simulink model "Time_Shift_1"  (R2015a)
settings: Solver=ode3  StartTime=0.0  StopTime=inf  FixedStep=.1  RelTol=1e-3
libraries: xpcutilitieslib x31, slrtlib x10, AAxpcseriallibold x9, xpcobsoletelib x5, etargetslib x1
settings Model: SimulationMode=external  Creator=farbod  LastModifiedBy=Darryl
settings SolverCC: EnableConcurrentExecution=on
settings DataIOCC: SignalLoggingSaveFormat=ModelDataLogs
settings OptimizationCC: BlockReduction=off  OptimizeBlockIOStorage=off  BufferReuse=off  GlobalBufferReuse=off  ExpressionFolding=off  ExpressionDepthLimit=2147483647  LocalBlockOutputs=off
settings DebuggingCC: UnderspecifiedInitializationDetection=Classic  MergeDetectMultiDrivingBlocksExec=none  FcnCallInpInsideContextMsg=UseLocalSettings  StateNameClashWarn=warning
settings HardwareCC: ProdIntDivRoundTo=Zero  ProdEndianess=LittleEndian  ProdLongLongMode=on  ProdHWDeviceType=Generic->32-bit x86 compatible  TargetBitPerLong=64  TargetBitPerPointer=64  TargetIntDivRoundTo=Zero  TargetEndianess=LittleEndian  TargetWordSize=64  TargetHWDeviceType=Intel->x86-64
settings SFSimCC: SimParseCustomCode=off
settings RTWCC: SystemTargetFile=slrt.tlc  TemplateMakefile=slrt_default_tmf  Description=Simulink Real-Time  RTWVerbose=off  RTWCompilerOptimization=on
settings CodeAppCC: MaxIdLength=95
settings SimulinkRealTimeCC: GeneratePreprocessorConditionals=Disable all

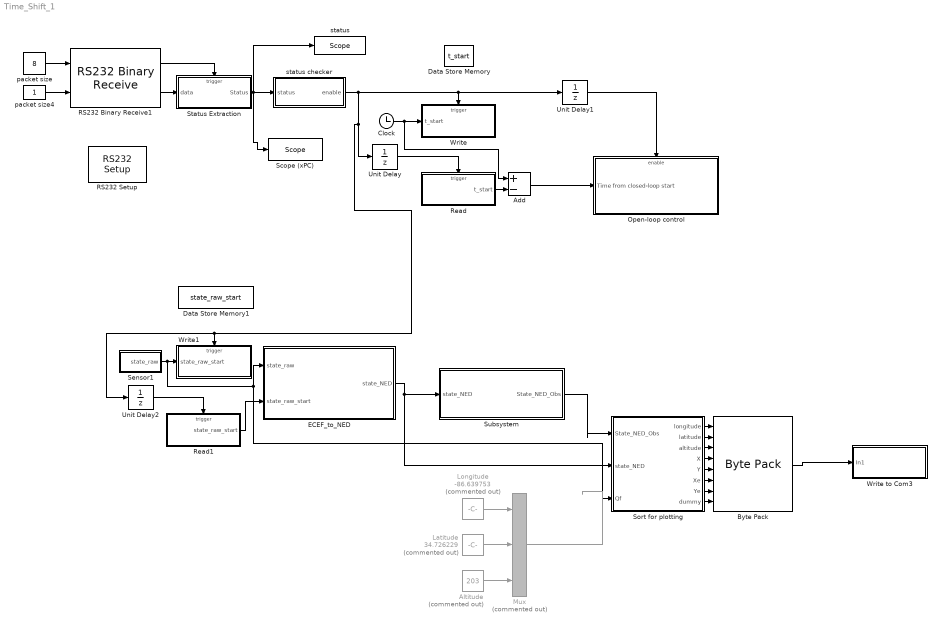
== system Time_Shift_1 ==
  Add : Sum  Inputs=+-
  Altitude : Constant  Commented=on  Value=203
  Byte Pack : etargetslib/Byte Pack  datatypes={'uint8','uint8','uint8','uint8','uint8','uint8','uint8','uint8'}  byteAlign=1
  Clock : Clock
  Data Store Memory : DataStoreMemory  DataStoreName=t_start  ReadBeforeWriteMsg=warning  WriteAfterWriteMsg=warning  WriteAfterReadMsg=warning
  Data Store Memory1 : DataStoreMemory  DataStoreName=state_raw_start  ReadBeforeWriteMsg=warning  WriteAfterWriteMsg=warning  WriteAfterReadMsg=warning  InitialValue=[-86.647163*pi/180;34.718727*pi/180;195;0;0;0;0;0;0;0;0;0;0;0;-1]
  ECEF_to_NED : MATLAB Function  TreatAsAtomicUnit=on
  Latitude : Constant  Commented=on  Value=34.726229
  Longitude : Constant  Commented=on  Value=-86.639753
  Mux : Mux  Commented=on  Inputs=3
  Open-loop control : Subsystem
  RS232 Binary Receive1 : AAxpcseriallibold/Obsolete/Binary Mode/RS232 Binary Receive  port=COM1  width=8  samptime=-1
  "RS232 Setup " : AAxpcseriallibold/Obsolete/RS232 Setup   port=COM1  baud=115200  dbits=8  sbits=1  parity=None  prot=None  sbuf=2048  rbuf=2048  initstruct=[]  termstruct=[]
  Read : Subsystem  TreatAsAtomicUnit=on
  Read1 : Subsystem  TreatAsAtomicUnit=on
  "Scope (xPC) " : slrtlib/Displays and Logging/Scope   scopeno=2  scopetype=Target  autostart=on  viewmode=Graphical rolling  formatstr='status=%3.3f'  grid=on  ylimits=[0,0]  nosamples=2000  noprepostsamples=0  interleave=1  triggermode=FreeRun  triggersignal=1  trigsignalfromport=off  triggerlevel=0.0  triggerslope=Either  triggerscope=1  triggersample=0  filename=data.dat  mode=Lazy  writesize=512  autorestart=off  dynamicfilemode=off  maxwritefilesize=512*1024^2
  Sensor1 : Subsystem
  Sort for plotting : MATLAB Function  TreatAsAtomicUnit=on
  Status Extraction : Subsystem  TreatAsAtomicUnit=on
  Subsystem : Subsystem
  Unit Delay : UnitDelay  SampleTime=-1
  Unit Delay1 : UnitDelay  SampleTime=-1
  Unit Delay2 : UnitDelay  SampleTime=-1
  Write : Subsystem  TreatAsAtomicUnit=on
  Write to Com3 : Subsystem
  Write1 : Subsystem  TreatAsAtomicUnit=on
  packet size : Constant  Value=8
  packet size4 : Constant
  status : slrtlib/Displays and Logging/Scope   scopeno=6  scopetype=File  autostart=on  viewmode=Graphical rolling  formatstr='%15.6f'  grid=on  ylimits=[-10,50]  nosamples=3000  noprepostsamples=0  interleave=1  triggermode=FreeRun  triggersignal=1  trigsignalfromport=off  triggerlevel=0.0  triggerslope=Either  triggerscope=1  triggersample=0  filename=1sttus01.dat  mode=Commit  writesize=512  autorestart=on  dynamicfilemode=off  maxwritefilesize=512*1024^2
  status checker : MATLAB Function  TreatAsAtomicUnit=on
  wires:
  Unit Delay/1 -> Read/Trigger
  Clock/1 -> Write/1(t_start), Add/1
  Read/1(t_start) -> Add/2
  Status Extraction/1(Status) -> status/1, "Scope (xPC) "/1, status checker/1(status)
  status checker/1(enable) -> Write/Trigger, Unit Delay1/1, Unit Delay/1, Unit Delay2/1, Write1/Trigger
  Unit Delay1/1 -> Open-loop control/Enable
  Add/1 -> Open-loop control/1(Time from closed-loop start)
  Sensor1/1(state_raw) -> Write1/1(state_raw_start), Sort for plotting/3(Qf), ECEF_to_NED/1(state_raw)
  Unit Delay2/1 -> Read1/Trigger
  Read1/1(state_raw_start) -> ECEF_to_NED/2(state_raw_start)
  ECEF_to_NED/1(state_NED) -> Sort for plotting/2(state_NED), Subsystem/1(state_NED)
  RS232 Binary Receive1/2 -> Status Extraction/1(data)
  RS232 Binary Receive1/1 -> Status Extraction/Trigger
  packet size4/1 -> RS232 Binary Receive1/2
  packet size/1 -> RS232 Binary Receive1/1
  Subsystem/1(State_NED_Obs) -> Sort for plotting/1(State_NED_Obs)
  Latitude/1 -> Mux/2
  Altitude/1 -> Mux/3
  Longitude/1 -> Mux/1
  Mux/1 -> ?
  Byte Pack/1 -> Write to Com3/1(In1)
  Sort for plotting/1(longitude) -> Byte Pack/1
  Sort for plotting/2(latitude) -> Byte Pack/2
  Sort for plotting/3(altitude) -> Byte Pack/3
  Sort for plotting/4(X) -> Byte Pack/4
  Sort for plotting/5(Y) -> Byte Pack/5
  Sort for plotting/6(Xe) -> Byte Pack/6
  Sort for plotting/7(Ye) -> Byte Pack/7
  Sort for plotting/8(dummy) -> Byte Pack/8

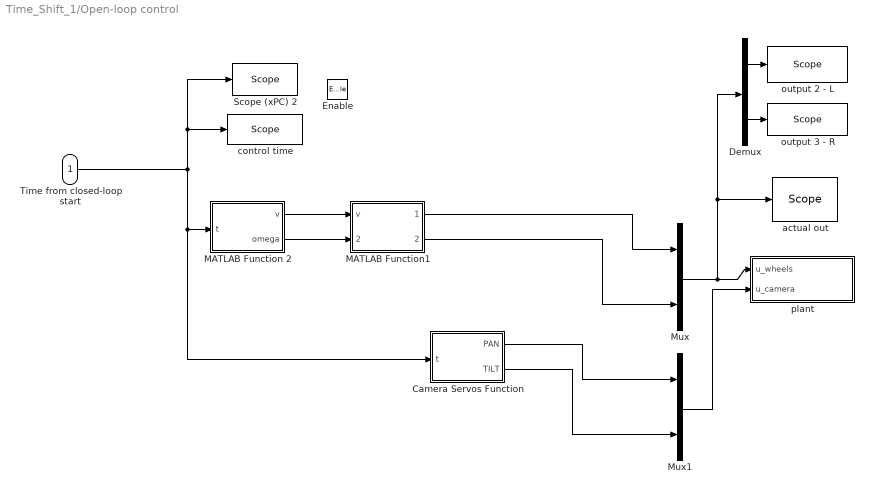
== system Time_Shift_1/Open-loop control ==
  Time from closed-loop start : Inport
  Enable : EnablePort  PropagateVarSize=During execution
  " MATLAB Function1" : MATLAB Function  TreatAsAtomicUnit=on
  Camera Servos Function : MATLAB Function  TreatAsAtomicUnit=on
  Demux : Demux  Outputs=2
  MATLAB Function 2 : MATLAB Function  TreatAsAtomicUnit=on
  Mux : Mux  Inputs=2
  Mux1 : Mux  Inputs=2
  Scope (xPC) 2 : slrtlib/Displays and Logging/Scope   scopeno=1  scopetype=File  autostart=on  viewmode=Graphical redraw  formatstr='%15.6f'  grid=on  ylimits=[0,0]  nosamples=3000  noprepostsamples=0  interleave=1  triggermode=FreeRun  triggersignal=1  trigsignalfromport=off  triggerlevel=0.0  triggerslope=Either  triggerscope=1  triggersample=0  filename=1ctime01.dat  mode=Commit  writesize=512  autorestart=off  dynamicfilemode=off  maxwritefilesize=512*1024^2
  actual out : slrtlib/Displays and Logging/Scope   scopeno=7  scopetype=File  autostart=on  viewmode=Graphical rolling  formatstr='%15.6f'  grid=on  ylimits=[-3,150]  nosamples=3000  noprepostsamples=0  interleave=1  triggermode=FreeRun  triggersignal=1  trigsignalfromport=off  triggerlevel=0.0  triggerslope=Either  triggerscope=1  triggersample=0  filename=1pwm01.dat  mode=Commit  writesize=512  autorestart=on  dynamicfilemode=off  maxwritefilesize=512*1024^2
  control time : slrtlib/Displays and Logging/Scope   scopeno=9  scopetype=Target  autostart=on  viewmode=Graphical rolling  formatstr='t=%3.3f'  grid=on  ylimits=[0,0]  nosamples=2000  noprepostsamples=0  interleave=1  triggermode=FreeRun  triggersignal=1  trigsignalfromport=off  triggerlevel=0.0  triggerslope=Either  triggerscope=1  triggersample=0  filename=data.dat  mode=Lazy  writesize=512  autorestart=off  dynamicfilemode=off  maxwritefilesize=512*1024^2
  output 2 - L : slrtlib/Displays and Logging/Scope   scopeno=10  scopetype=Target  autostart=on  viewmode=Graphical rolling  formatstr='u1=%3.3f'  grid=on  ylimits=[0,0]  nosamples=20000  noprepostsamples=0  interleave=1  triggermode=FreeRun  triggersignal=1  trigsignalfromport=off  triggerlevel=0.0  triggerslope=Either  triggerscope=1  triggersample=0  filename=data.dat  mode=Lazy  writesize=512  autorestart=off  dynamicfilemode=off  maxwritefilesize=512*1024^2
  output 3 - R : slrtlib/Displays and Logging/Scope   scopeno=5  scopetype=Target  autostart=on  viewmode=Graphical rolling  formatstr='u2=%3.3f'  grid=on  ylimits=[0,0]  nosamples=20000  noprepostsamples=0  interleave=1  triggermode=FreeRun  triggersignal=1  trigsignalfromport=off  triggerlevel=0.0  triggerslope=Either  triggerscope=1  triggersample=0  filename=data.dat  mode=Lazy  writesize=512  autorestart=off  dynamicfilemode=off  maxwritefilesize=512*1024^2
  plant : Subsystem
  wires:
  Time from closed-loop start/1 -> control time/1, Scope (xPC) 2/1, MATLAB Function 2/1(t), Camera Servos Function/1(t)
  Demux/1 -> output 2 - L/1
  Demux/2 -> output 3 - R/1
  Mux/1 -> plant/1(u_wheels), actual out/1, Demux/1
  MATLAB Function 2/1(v) -> " MATLAB Function1"/1(v)
  MATLAB Function 2/2(omega) -> " MATLAB Function1"/2(omega)
  " MATLAB Function1"/1(PWM_L) -> Mux/1
  " MATLAB Function1"/2(PWM_R) -> Mux/2
  Camera Servos Function/1(PAN) -> Mux1/1
  Camera Servos Function/2(TILT) -> Mux1/2
  Mux1/1 -> plant/2(u_camera)

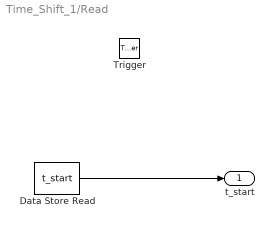
== system Time_Shift_1/Read ==
  Trigger : TriggerPort
  Data Store Read : DataStoreRead  DataStoreName=t_start
  t_start : Outport
  wires:
  Data Store Read/1 -> t_start/1

== system Time_Shift_1/Read1 ==
  Trigger : TriggerPort
  Data Store Read : DataStoreRead  DataStoreName=state_raw_start
  state_raw_start : Outport
  wires:
  Data Store Read/1 -> state_raw_start/1

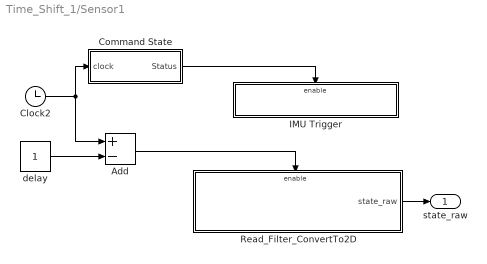
== system Time_Shift_1/Sensor1 ==
  Add : Sum  Inputs=+-
  Clock2 : Clock
  Command State : MATLAB Function  TreatAsAtomicUnit=on
  IMU Trigger : Subsystem
  Read_Filter_ConvertTo2D : Subsystem
  delay : Constant
  state_raw : Outport
  wires:
  Clock2/1 -> Add/1, Command State/1(clock)
  Read_Filter_ConvertTo2D/1(state_raw) -> state_raw/1
  delay/1 -> Add/2
  Add/1 -> Read_Filter_ConvertTo2D/Enable
  Command State/1(Status) -> IMU Trigger/Enable

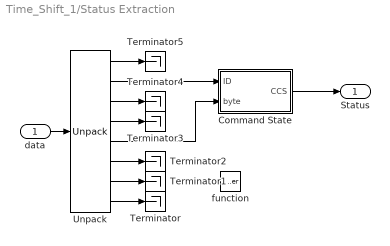
== system Time_Shift_1/Status Extraction ==
  data : Inport
  function : TriggerPort  TriggerType=function-call  OutputDataType=int8
  Command State : MATLAB Function  TreatAsAtomicUnit=on
  Terminator{,1..5} (6 alike) : Terminator
  Unpack : xpcobsoletelib/Utilities/Unpack   dimensions={1,1,1,1,1,1,1,1}  datatypes={'uint8','uint8','uint8','uint8','uint8','uint8','uint8','uint8'}  byteAlign=1
  Status : Outport
  wires:
  data/1 -> Unpack/1
  Command State/1(CCS) -> Status/1
  Unpack/5 -> Command State/2(byte)
  Unpack/2 -> Command State/1(ID)
  Unpack/8 -> Terminator/1
  Unpack/1 -> Terminator5/1
  Unpack/3 -> Terminator4/1
  Unpack/4 -> Terminator3/1
  Unpack/6 -> Terminator2/1
  Unpack/7 -> Terminator1/1

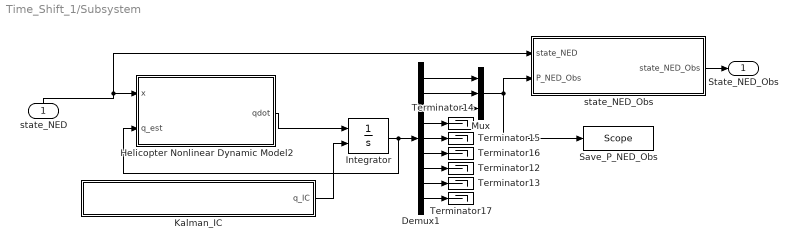
== system Time_Shift_1/Subsystem ==
  state_NED : Inport
  Demux1 : Demux  Outputs=9
  Helicopter Nonlinear Dynamic Model2 : MATLAB Function  TreatAsAtomicUnit=on
  Integrator : Integrator  InitialConditionSource=external
  Kalman_IC : MATLAB Function  TreatAsAtomicUnit=on
  Mux : Mux  Inputs=3
  Save_P_NED_Obs : slrtlib/Displays and Logging/Scope   scopeno=4  scopetype=File  autostart=on  viewmode=Graphical rolling  formatstr='%15.6f'  grid=on  ylimits=[-10,50]  nosamples=3000  noprepostsamples=0  interleave=1  triggermode=FreeRun  triggersignal=1  trigsignalfromport=off  triggerlevel=0.0  triggerslope=Either  triggerscope=1  triggersample=0  filename=1P_NED1.dat  mode=Commit  writesize=512  autorestart=on  dynamicfilemode=off  maxwritefilesize=512*1024^2
  Terminator{12..17} (6 alike) : Terminator
  state_NED_Obs : MATLAB Function  TreatAsAtomicUnit=on
  State_NED_Obs : Outport
  wires:
  state_NED/1 -> state_NED_Obs/1(state_NED), Helicopter Nonlinear Dynamic Model2/1(x)
  Integrator/1 -> Demux1/1, Helicopter Nonlinear Dynamic Model2/2(q_est)
  Kalman_IC/1(q_IC) -> Integrator/2
  Demux1/4 -> Terminator14/1
  Demux1/5 -> Terminator15/1
  Demux1/6 -> Terminator16/1
  Demux1/7 -> Terminator12/1
  Demux1/8 -> Terminator13/1
  Demux1/9 -> Terminator17/1
  Helicopter Nonlinear Dynamic Model2/1(qdot) -> Integrator/1
  Demux1/3 -> Mux/3
  Demux1/2 -> Mux/2
  Demux1/1 -> Mux/1
  Mux/1 -> state_NED_Obs/2(P_NED_Obs), Save_P_NED_Obs/1
  state_NED_Obs/1(state_NED_Obs) -> State_NED_Obs/1

== system Time_Shift_1/Write ==
  t_start : Inport
  Trigger : TriggerPort
  Data Store Write : DataStoreWrite  DataStoreName=t_start
  wires:
  t_start/1 -> Data Store Write/1

== system Time_Shift_1/Write to Com3 ==
  In1 : Inport
  RS232 Binary Send : AAxpcseriallibold/Obsolete/Binary Mode/RS232 Binary Send  port=COM3  width=64  samptime=-1
  "RS232 Setup " : AAxpcseriallibold/Obsolete/RS232 Setup   port=COM3  baud=19200  dbits=8  sbits=1  parity=None  prot=XOn XOff  sbuf=960000  rbuf=2048  initstruct=[]  termstruct=[]
  wires:
  In1/1 -> RS232 Binary Send/1

== system Time_Shift_1/Write1 ==
  state_raw_start : Inport
  Trigger : TriggerPort
  Data Store Write : DataStoreWrite  DataStoreName=state_raw_start
  wires:
  state_raw_start/1 -> Data Store Write/1

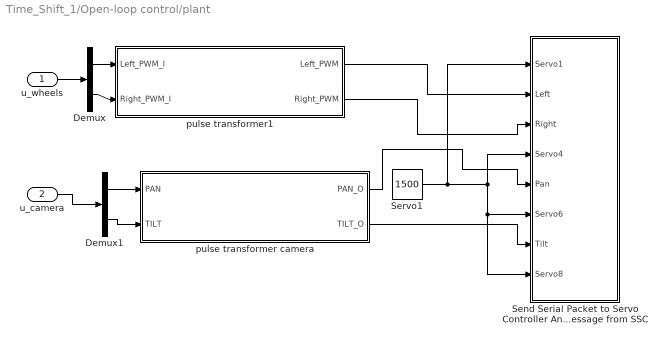
== system Time_Shift_1/Open-loop control/plant ==
  u_wheels : Inport
  u_camera : Inport  Port=2
  Demux : Demux  Outputs=2
  Demux1 : Demux  Outputs=2
  Send Serial Packet to Servo Controller And recieve status message from SSC : Subsystem  TreatAsAtomicUnit=on
  Servo1 : Constant  Value=1500  OutDataTypeStr=uint16
  pulse transformer camera : MATLAB Function  TreatAsAtomicUnit=on
  pulse transformer1 : MATLAB Function  TreatAsAtomicUnit=on
  wires:
  Servo1/1 -> Send Serial Packet to Servo Controller And recieve status message from SSC/6(Servo6), Send Serial Packet to Servo Controller And recieve status message from SSC/8(Servo8), Send Serial Packet to Servo Controller And recieve status message from SSC/4(Servo4), Send Serial Packet to Servo Controller And recieve status message from SSC/1(Servo1)
  u_wheels/1 -> Demux/1
  Demux/1 -> pulse transformer1/1(Left_PWM_I)
  Demux/2 -> pulse transformer1/2(Right_PWM_I)
  u_camera/1 -> Demux1/1
  pulse transformer1/1(Left_PWM) -> Send Serial Packet to Servo Controller And recieve status message from SSC/2(Left)
  pulse transformer1/2(Right_PWM) -> Send Serial Packet to Servo Controller And recieve status message from SSC/3(Right)
  Demux1/1 -> pulse transformer camera/1(PAN)
  Demux1/2 -> pulse transformer camera/2(TILT)
  pulse transformer camera/1(PAN_O) -> Send Serial Packet to Servo Controller And recieve status message from SSC/5(Pan)
  pulse transformer camera/2(TILT_O) -> Send Serial Packet to Servo Controller And recieve status message from SSC/7(Tilt)

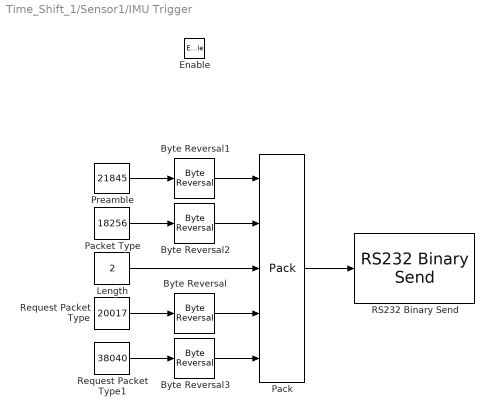
== system Time_Shift_1/Sensor1/IMU Trigger ==
  Enable : EnablePort  PropagateVarSize=During execution
  Byte Reversal{,1..3} (4 alike) : xpcutilitieslib/Byte Reversal   numInp=1
  Length : Constant  Value=2  OutDataTypeStr=uint8
  Pack : xpcobsoletelib/Utilities/Pack   datatypes={'uint16','uint16','uint8','uint16','uint16'}  byteAlign=1
  Packet Type : Constant  Value=18256  OutDataTypeStr=uint16
  Preamble : Constant  Value=21845  OutDataTypeStr=uint16
  RS232 Binary Send : AAxpcseriallibold/Obsolete/Binary Mode/RS232 Binary Send  port=COM2  width=9  samptime=-1
  Request Packet Type : Constant  Value=20017  OutDataTypeStr=uint16
  Request Packet Type1 : Constant  Value=38040  OutDataTypeStr=uint16
  wires:
  Pack/1 -> RS232 Binary Send/1
  Preamble/1 -> Byte Reversal1/1
  Packet Type/1 -> Byte Reversal2/1
  Length/1 -> Pack/3
  Request Packet Type/1 -> Byte Reversal/1
  Request Packet Type1/1 -> Byte Reversal3/1
  Byte Reversal/1 -> Pack/4
  Byte Reversal1/1 -> Pack/1
  Byte Reversal2/1 -> Pack/2
  Byte Reversal3/1 -> Pack/5

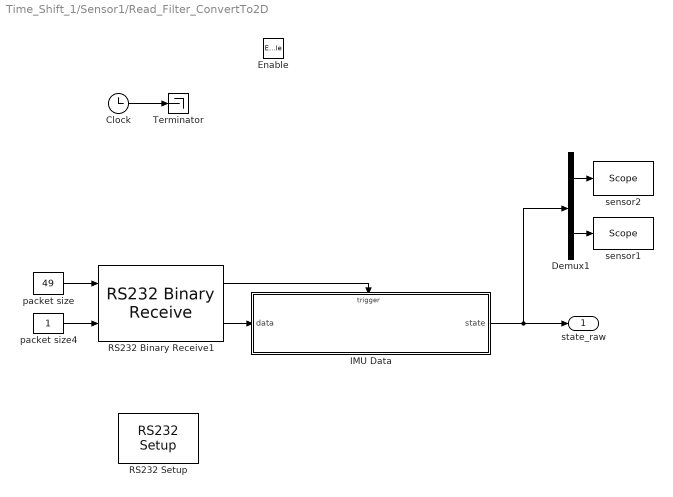
== system Time_Shift_1/Sensor1/Read_Filter_ConvertTo2D ==
  Enable : EnablePort  PropagateVarSize=During execution
  Clock : Clock
  Demux1 : Demux  Outputs=2
  IMU Data : Subsystem  TreatAsAtomicUnit=on
  RS232 Binary Receive1 : AAxpcseriallibold/Obsolete/Binary Mode/RS232 Binary Receive  port=COM2  width=49  samptime=-1
  "RS232 Setup " : AAxpcseriallibold/Obsolete/RS232 Setup   port=COM2  baud=57600  dbits=8  sbits=1  parity=None  prot=None  sbuf=1024  rbuf=1024  initstruct=[]  termstruct=[]
  Terminator : Terminator
  packet size : Constant  Value=49
  packet size4 : Constant
  sensor1 : slrtlib/Displays and Logging/Scope   scopeno=8  scopetype=File  autostart=on  viewmode=Graphical rolling  formatstr='%15.6f'  grid=on  ylimits=[-10,50]  nosamples=3000  noprepostsamples=0  interleave=1  triggermode=FreeRun  triggersignal=1  trigsignalfromport=off  triggerlevel=0.0  triggerslope=Either  triggerscope=1  triggersample=0  filename=1sens12.dat  mode=Commit  writesize=512  autorestart=on  dynamicfilemode=off  maxwritefilesize=512*1024^2
  sensor2 : slrtlib/Displays and Logging/Scope   scopeno=11  scopetype=File  autostart=on  viewmode=Graphical rolling  formatstr='%15.6f'  grid=on  ylimits=[-10,50]  nosamples=3000  noprepostsamples=0  interleave=1  triggermode=FreeRun  triggersignal=1  trigsignalfromport=off  triggerlevel=0.0  triggerslope=Either  triggerscope=1  triggersample=0  filename=1sens13.dat  mode=Commit  writesize=512  autorestart=on  dynamicfilemode=off  maxwritefilesize=512*1024^2
  state_raw : Outport
  wires:
  Demux1/2 -> sensor1/1
  Demux1/1 -> sensor2/1
  Clock/1 -> Terminator/1
  packet size/1 -> RS232 Binary Receive1/1
  packet size4/1 -> RS232 Binary Receive1/2
  IMU Data/1(state) -> Demux1/1, state_raw/1
  RS232 Binary Receive1/2 -> IMU Data/1(data)
  RS232 Binary Receive1/1 -> IMU Data/Trigger

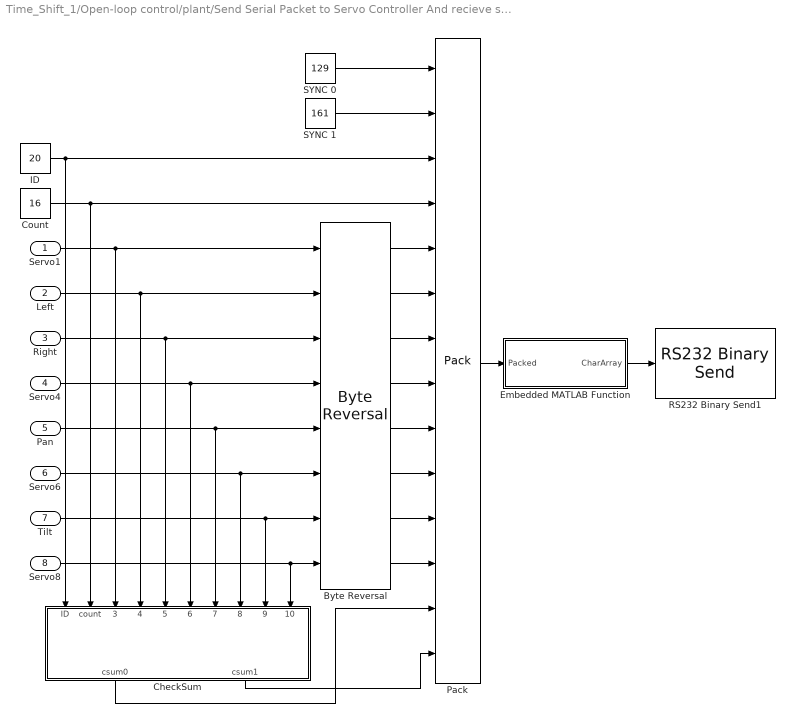
== system Time_Shift_1/Open-loop control/plant/Send Serial Packet to Servo Controller And recieve status message from SSC ==
  Servo1 : Inport  OutDataTypeStr=uint16
  Left : Inport  Port=2  OutDataTypeStr=uint16
  Right : Inport  Port=3  OutDataTypeStr=uint16
  Servo4 : Inport  Port=4  OutDataTypeStr=uint16
  Pan : Inport  Port=5  OutDataTypeStr=uint16
  Servo6 : Inport  Port=6  OutDataTypeStr=uint16
  Tilt : Inport  Port=7  OutDataTypeStr=uint16
  Servo8 : Inport  Port=8  OutDataTypeStr=uint16
  Byte Reversal : xpcutilitieslib/Byte Reversal   numInp=8
  CheckSum : MATLAB Function  TreatAsAtomicUnit=on
  Count : Constant  Value=16  OutDataTypeStr=uint8
  Embedded MATLAB Function : MATLAB Function  TreatAsAtomicUnit=on
  ID : Constant  Value=20  OutDataTypeStr=uint8
  Pack : xpcobsoletelib/Utilities/Pack   datatypes={'uint8','uint8','uint8','uint8','uint16','uint16','uint16','uint16','uint16','uint16','uint16','uint16','uint8','uint8'}  byteAlign=1
  RS232 Binary Send1 : AAxpcseriallibold/Obsolete/Binary Mode/RS232 Binary Send  port=COM1  width=22  samptime=-1
  SYNC 0 : Constant  Value=129  OutDataTypeStr=uint8
  SYNC 1 : Constant  Value=161  OutDataTypeStr=uint8
  wires:
  SYNC 0/1 -> Pack/1
  SYNC 1/1 -> Pack/2
  ID/1 -> Pack/3, CheckSum/1(ID)
  Count/1 -> Pack/4, CheckSum/2(count)
  Byte Reversal/2 -> Pack/6
  Byte Reversal/1 -> Pack/5
  Byte Reversal/3 -> Pack/7
  Byte Reversal/4 -> Pack/8
  Byte Reversal/5 -> Pack/9
  Byte Reversal/6 -> Pack/10
  Byte Reversal/7 -> Pack/11
  Byte Reversal/8 -> Pack/12
  CheckSum/2(csum1) -> Pack/14
  CheckSum/1(csum0) -> Pack/13
  Servo8/1 -> Byte Reversal/8, CheckSum/10(servo8)
  Tilt/1 -> Byte Reversal/7, CheckSum/9(servo7)
  Servo6/1 -> Byte Reversal/6, CheckSum/8(servo6)
  Pan/1 -> Byte Reversal/5, CheckSum/7(servo5)
  Servo4/1 -> Byte Reversal/4, CheckSum/6(servo4)
  Right/1 -> Byte Reversal/3, CheckSum/5(servo3)
  Left/1 -> Byte Reversal/2, CheckSum/4(servo2)
  Servo1/1 -> Byte Reversal/1, CheckSum/3(servo1)
  Pack/1 -> Embedded MATLAB Function/1(Packed)
  Embedded MATLAB Function/1(CharArray) -> RS232 Binary Send1/1

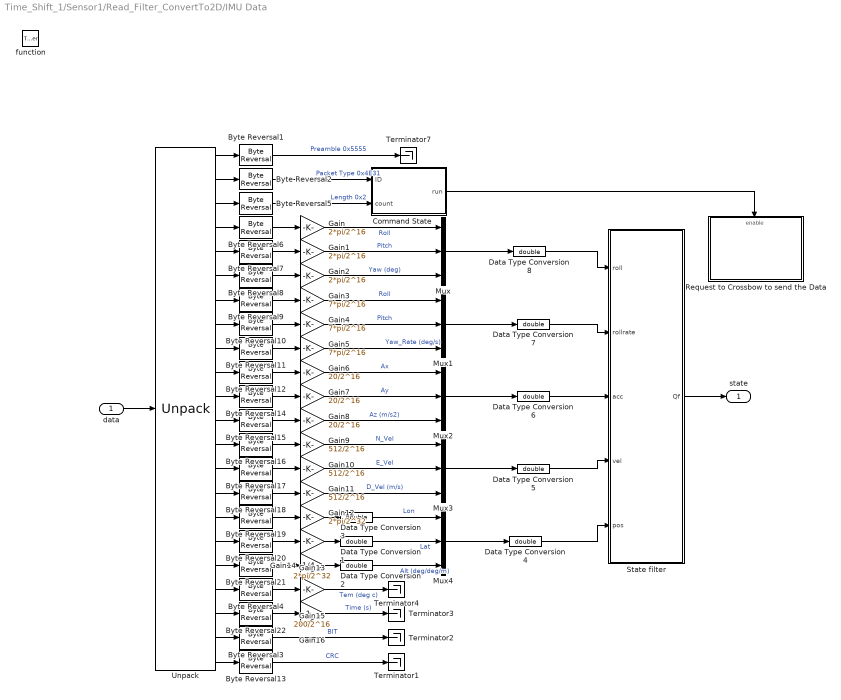
== system Time_Shift_1/Sensor1/Read_Filter_ConvertTo2D/IMU Data ==
  data : Inport
  function : TriggerPort  TriggerType=function-call  OutputDataType=int8
  Byte Reversal{1..22} (22 alike) : xpcutilitieslib/Byte Reversal   numInp=1
  Command State : MATLAB Function  TreatAsAtomicUnit=on
  Data Type Conversion{1..8} (8 alike) : DataTypeConversion  OutDataTypeStr=double
  Gain : Gain  Gain=2*pi/2^16
  Gain1 : Gain  Gain=2*pi/2^16
  Gain10 : Gain  Gain=512/2^16
  Gain11 : Gain  Gain=512/2^16
  Gain12 : Gain  Gain=2*pi/2^32
  Gain13 : Gain  Gain=2*pi/2^32
  Gain14 : Gain  Gain=1/4
  Gain15 : Gain  Gain=200/2^16
  Gain16 : Gain
  Gain2 : Gain  Gain=2*pi/2^16
  Gain3 : Gain  Gain=7*pi/2^16
  Gain4 : Gain  Gain=7*pi/2^16
  Gain5 : Gain  Gain=7*pi/2^16
  Gain6 : Gain  Gain=20/2^16
  Gain7 : Gain  Gain=20/2^16
  Gain8 : Gain  Gain=20/2^16
  Gain9 : Gain  Gain=512/2^16
  Mux{,1..4} (5 alike) : Mux  Inputs=3
  Request to Crossbow to send the Data : Subsystem
  State filter : MATLAB Function  TreatAsAtomicUnit=on
  Terminator{1..4,7} (5 alike) : Terminator
  Unpack : xpcobsoletelib/Utilities/Unpack   dimensions={1,1,1,1,1,1,1,1,1,1,1,1,1,1,1,1,1,1,1,1,1,1}  datatypes={'uint16','uint16','uint8','int16','int16','int16','int16','int16','int16','int16','int16','int16','int16','int16','int16','int32','int32','int16','int16','uint32','uint16','uint16'}  byteAlign=1
  state : Outport
  wires:
  data/1 -> Unpack/1
  Unpack/1 -> Byte Reversal1/1
  Unpack/2 -> Byte Reversal2/1
  Unpack/3 -> Byte Reversal5/1
  Unpack/4 -> Byte Reversal6/1
  Unpack/5 -> Byte Reversal7/1
  Unpack/6 -> Byte Reversal8/1
  Unpack/7 -> Byte Reversal9/1
  Unpack/8 -> Byte Reversal10/1
  Byte Reversal1/1 -> Terminator7/1  "Preamble 0x5555"
  Byte Reversal2/1 -> Command State/1(ID)  "Packet Type 0x4E31"
  Command State/1(run) -> Request to Crossbow to send the Data/Enable
  Unpack/21 -> Byte Reversal3/1
  Unpack/19 -> Byte Reversal4/1
  Byte Reversal5/1 -> Command State/2(count)  "Length 0x2"
  Byte Reversal9/1 -> Gain3/1
  Byte Reversal10/1 -> Gain4/1
  Byte Reversal6/1 -> Gain/1
  Byte Reversal7/1 -> Gain1/1
  Byte Reversal8/1 -> Gain2/1
  Gain/1 -> Mux/1  "Roll"
  Gain1/1 -> Mux/2  "Pitch"
  Gain2/1 -> Mux/3  "Yaw (deg)"
  Gain3/1 -> Mux1/1  "Roll"
  Gain4/1 -> Mux1/2  "Pitch"
  Unpack/9 -> Byte Reversal11/1
  Byte Reversal11/1 -> Gain5/1
  Gain5/1 -> Mux1/3  "Yaw_Rate (deg/s)"
  Gain6/1 -> Mux2/1  "Ax"
  Byte Reversal12/1 -> Gain6/1
  Unpack/10 -> Byte Reversal12/1
  Mux/1 -> Data Type Conversion8/1
  Unpack/22 -> Byte Reversal13/1
  Byte Reversal3/1 -> Terminator2/1  "BIT"
  Byte Reversal13/1 -> Terminator1/1  "CRC"
  Unpack/20 -> Byte Reversal22/1
  Mux1/1 -> Data Type Conversion7/1
  Mux2/1 -> Data Type Conversion6/1
  Byte Reversal14/1 -> Gain7/1
  Byte Reversal15/1 -> Gain8/1
  Unpack/11 -> Byte Reversal14/1
  Unpack/12 -> Byte Reversal15/1
  Gain7/1 -> Mux2/2  "Ay"
  Gain8/1 -> Mux2/3  "Az (m/s2)"
  Mux3/1 -> Data Type Conversion5/1
  Unpack/13 -> Byte Reversal16/1
  Byte Reversal16/1 -> Gain9/1
  Byte Reversal17/1 -> Gain10/1
  Byte Reversal18/1 -> Gain11/1
  Unpack/14 -> Byte Reversal17/1
  Unpack/15 -> Byte Reversal18/1
  Gain9/1 -> Mux3/1  "N_Vel"
  Gain10/1 -> Mux3/2  "E_Vel"
  Gain11/1 -> Mux3/3  "D_Vel (m/s)"
  Unpack/16 -> Byte Reversal19/1
  Unpack/17 -> Byte Reversal20/1
  Unpack/18 -> Byte Reversal21/1
  Byte Reversal20/1 -> Gain13/1
  Byte Reversal19/1 -> Gain12/1
  Mux4/1 -> Data Type Conversion4/1
  Gain12/1 -> Data Type Conversion3/1
  Gain13/1 -> Data Type Conversion1/1
  Gain14/1 -> Data Type Conversion2/1
  Byte Reversal21/1 -> Gain14/1
  Byte Reversal22/1 -> Gain16/1
  Byte Reversal4/1 -> Gain15/1
  Gain15/1 -> Terminator4/1  "Tem (deg c)"
  Gain16/1 -> Terminator3/1  "Time (s)"
  Data Type Conversion2/1 -> Mux4/3  "Alt (deg/deg/m)"
  Data Type Conversion1/1 -> Mux4/2  "Lat"
  Data Type Conversion3/1 -> Mux4/1  "Lon"
  State filter/1(Qf) -> state/1
  Data Type Conversion4/1 -> State filter/5(pos)
  Data Type Conversion5/1 -> State filter/4(vel)
  Data Type Conversion6/1 -> State filter/3(acc)
  Data Type Conversion7/1 -> State filter/2(rollrate)
  Data Type Conversion8/1 -> State filter/1(roll)

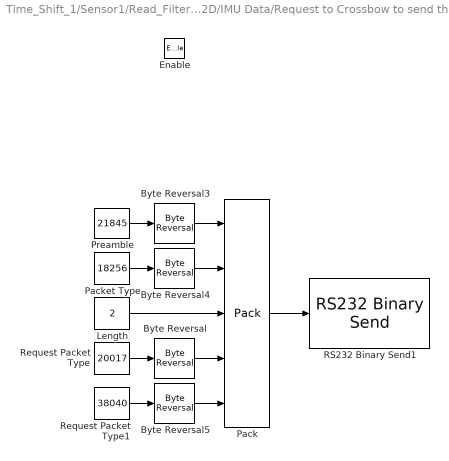
== system Time_Shift_1/Sensor1/Read_Filter_ConvertTo2D/IMU Data/Request to Crossbow to send the Data ==
  Enable : EnablePort  PropagateVarSize=During execution
  Byte Reversal{,3..5} (4 alike) : xpcutilitieslib/Byte Reversal   numInp=1
  Length : Constant  Value=2  OutDataTypeStr=uint8
  Pack : xpcobsoletelib/Utilities/Pack   datatypes={'uint16','uint16','uint8','uint16','uint16'}  byteAlign=1
  Packet Type : Constant  Value=18256  OutDataTypeStr=uint16
  Preamble : Constant  Value=21845  OutDataTypeStr=uint16
  RS232 Binary Send1 : AAxpcseriallibold/Obsolete/Binary Mode/RS232 Binary Send  port=COM2  width=9  samptime=-1
  Request Packet Type : Constant  Value=20017  OutDataTypeStr=uint16
  Request Packet Type1 : Constant  Value=38040  OutDataTypeStr=uint16
  wires:
  Pack/1 -> RS232 Binary Send1/1
  Preamble/1 -> Byte Reversal3/1
  Packet Type/1 -> Byte Reversal4/1
  Length/1 -> Pack/3
  Request Packet Type/1 -> Byte Reversal/1
  Request Packet Type1/1 -> Byte Reversal5/1
  Byte Reversal/1 -> Pack/4
  Byte Reversal3/1 -> Pack/1
  Byte Reversal4/1 -> Pack/2
  Byte Reversal5/1 -> Pack/5

== matlab function Time_Shift_1/Open-loop control/MATLAB Function 2 ==
  data: t input; v output; omega output
function [v,omega] = fcn(t)
%#codegen

tau = 10;

v0 = 0.9;
omega0 = 0.5;

tshift = 1;

v = v0*sin(2*pi*t/tau);
omega = omega0*sin(2*pi*(t-tshift)/tau);

== matlab function Time_Shift_1/Sensor1/Read_Filter_ConvertTo2D/IMU Data/State filter ==
  data: roll input; Qf output; rollrate input; acc input; vel input; pos input
function Qf = fcn( roll, rollrate, acc, vel, pos)
% This block supports an embeddable subset of the MATLAB language.
% See the help menu for details. 

% info is extracted from sensor
rol=roll(1);
pit=roll(2);
yaw=roll(3);
rollp=rollrate(1);
pitp=rollrate(2);
yawp=rollrate(3);
lon=pos(1);
lat=pos(2);
alt=pos(3);
vN=vel(1);
vE=vel(2);
vD=vel(3);
ax=acc(1);
ay=acc(2);
az=acc(3);

Qf = [lon;lat;alt;rol;pit;yaw;vN;vE;vD;rollp;pitp;yawp;ax;ay;az];

== matlab function Time_Shift_1/Open-loop control/plant/Send Serial Packet to Servo Controller And recieve status message from SSC/CheckSum ==
  data: ID input; csum0 output; count input; servo1 input; servo2 input; csum1 output; servo3 input; servo4 input; servo5 input; servo6 input; servo7 input; servo8 input
function [csum0,csum1]= fcn(ID,count,servo1,servo2,servo3,servo4,servo5,servo6,servo7,servo8)
% The purpose of this function is to calculate the fletcher checksum values
% as defined in internet RFC 1145
% See page 11 of the Microbotics Servo Switch/Controller Users Manual for 
% more information

% break into bytes
servo1a=uint8(bitshift(servo1,-8)); servo1b=uint8(servo1-uint16(servo1a)*256);
servo2a=uint8(bitshift(servo2,-8)); servo2b=uint8(servo2-uint16(servo2a)*256);
servo3a=uint8(bitshift(servo3,-8)); servo3b=uint8(servo3-uint16(servo3a)*256);
servo4a=uint8(bitshift(servo4,-8)); servo4b=uint8(servo4-uint16(servo4a)*256);
servo5a=uint8(bitshift(servo5,-8)); servo5b=uint8(servo5-uint16(servo5a)*256);
servo6a=uint8(bitshift(servo6,-8)); servo6b=uint8(servo6-uint16(servo6a)*256);
servo7a=uint8(bitshift(servo7,-8)); servo7b=uint8(servo7-uint16(servo7a)*256);
servo8a=uint8(bitshift(servo8,-8)); servo8b=uint8(servo8-uint16(servo8a)*256);
byte=[ID, count, servo1a, servo1b, servo2a, servo2b, servo3a, servo3b, servo4a, servo4b, servo5a, servo5b, servo6a, servo6b, servo7a, servo7b, servo8a, servo8b];

cksum0=uint16(0);cksum1=uint16(0); % initialize to zero
for i=1:(count+2)
    cksum0=mod((cksum0+uint16(byte(i))),256);
    cksum1=mod((cksum1+cksum0),256);
end

csum0=uint8(cksum0); csum1=uint8(cksum1);

== matlab function Time_Shift_1/Open-loop control/ MATLAB Function1 ==
  data: v input; PWM_L output; omega input; PWM_R output
function [PWM_L,PWM_R] = fcn(v,omega)
%#codegen

T = 0.42;

vL = v +(T/2)*omega;
vR = v -(T/2)*omega;

vVec = [vL;vR];

aL = 3.8863614532;
bL = -0.0026808274;

aR = 3.2707294485;
bR = -0.0022447804;

A = [aL;aR];
B = [[bL,0];[0,bR]];

PWM = (B)\(vVec-A);

PWM_L = PWM(1);
PWM_R = PWM(2);

== matlab function Time_Shift_1/Sensor1/Command State ==
  data: clock input; Status output
function Status = fcn(clock)

% Initialization:

if clock == 0
    out = 1;
else
    out = 0;
end
Status = out;

== matlab function Time_Shift_1/Sensor1/Read_Filter_ConvertTo2D/IMU Data/Command State ==
  data: ID input; count input; run output
function run = fcn(ID,count)

% In this program the signal ID and count will be checked 
% for the reliability of the data.

if count==42
    if ID==20017
        run=1;
    else
        run=0;
    end
else
    run=0;
end

== matlab function Time_Shift_1/ECEF_to_NED ==
  data: state_raw input; state_NED output; state_raw_start input
function state_NED  = GEO_to_NED(state_raw,state_raw_start)
%#eml

p0 = state_raw_start(1);
T0 = state_raw_start(2);
r0 = state_raw_start(3);

p = state_raw(1);
T = state_raw(2);
r = state_raw(3);

R   = 6378.137e3;
e_2 = 6.6943799014e-3;

NofT0 = R/sqrt(1-e_2*sin(T0)^2);

X_ECFE0=(r0+NofT0)*cos(T0)*cos(p0);
Y_ECFE0=(r0+NofT0)*cos(T0)*sin(p0);
Z_ECFE0=(r0+NofT0*(1-e_2))*sin(T0);

NofT = R/sqrt(1-e_2*sin(T)^2);

X_ECFE=(r+NofT)*cos(T)*cos(p);
Y_ECFE=(r+NofT)*cos(T)*sin(p);
Z_ECFE=(r+NofT*(1-e_2))*sin(T);

R_ECFE_to_NED=[-sin(T0)*cos(p0) -sin(T0)*sin(p0) cos(T0); -sin(p0) cos(p0) 0; -cos(T0)*cos(p0) -cos(T0)*sin(p0) -sin(T0)];

P_ECFE =[X_ECFE;Y_ECFE;Z_ECFE];
P_ECFE0=[X_ECFE0;Y_ECFE0;Z_ECFE0];

P_NED=R_ECFE_to_NED*(P_ECFE-P_ECFE0);

state_NED = [P_NED(1);P_NED(2);P_NED(3);state_raw(4);state_raw(5);state_raw(6);state_raw(7);state_raw(8);...
    state_raw(9);state_raw(10);state_raw(11);state_raw(12);state_raw(13);state_raw(14);state_raw(15)];

== matlab function Time_Shift_1/Subsystem/Helicopter Nonlinear Dynamic Model2 ==
  data: x input; qdot output; q_est input
function qdot=KalmanObs(x,q_est)

%%%%%%%%%%%%%%%%%%%% Helicopter Blade Aerodynamic Code %%%%%%%%%%%%%%%%%%%%
% Sepehr Pourrezaei Khaligh                                 Jul. 13, 2012 %
% Farbod Fahimi                                             Apr. 14, 2014 %
%%%%%%%%%%%%%%%%%%%%%%%%%%%%%%%%%%%%%%%%%%%%%%%%%%%%%%%%%%%%%%%%%%%%%%%%%%%

%q_est = [x_NED;y_NED;z_NED;vx_NED;vy_NED;vz_NED;ax_NED;ay_NED;az_NED];
%u = [x_NED;y_NED;z_NED;ax_NED;ay_NED;az_NED];
phi =   x(4); %roll
theta = x(5); %pitch
psi =   x(6); % yaw

g = 9.8066;

Rb2i = [cos(theta)*cos(psi),-cos(phi)*sin(psi)+sin(phi)*sin(theta)*cos(psi),sin(phi)*sin(psi)+cos(phi)*sin(theta)*cos(psi);cos(theta)*sin(psi),cos(phi)*cos(psi)+sin(phi)*sin(theta)*sin(psi),-sin(phi)*cos(psi)+cos(phi)*sin(theta)*sin(psi);-sin(theta),sin(phi)*cos(theta),cos(phi)*cos(theta)];

a_NED = Rb2i*[x(13);x(14);x(15)]*g+[0;0;1]*g;

u = [x(1);x(2);x(3);a_NED(1);a_NED(2);a_NED(3)];

A = [-4.1562         0         0    1.0000         0         0   -0.0938         0         0;
           0   -4.1562         0         0    1.0000         0         0   -0.0938         0;
           0         0   -4.3899         0         0    1.0000         0         0   -0.0779;
     -9.0771         0         0         0         0         0    0.4196         0         0;
           0   -9.0771         0         0         0         0         0    0.4196         0;
           0         0   -9.9391         0         0         0         0         0    0.1102;
     -9.3826         0         0         0         0         0   -2.0297         0         0;
           0   -9.3826         0         0         0         0         0   -2.0297         0;
           0         0   -7.7930         0         0         0         0         0   -7.0280];
       
B =  [4.1562         0         0    0.0938         0         0;
           0    4.1562         0         0    0.0938         0;
           0         0    4.3899         0         0    0.0779;
      9.0771         0         0    0.5804         0         0;
           0    9.0771         0         0    0.5804         0;
           0         0    9.9391         0         0    0.8898;
      9.3826         0         0    2.0297         0         0;
           0    9.3826         0         0    2.0297         0;
           0         0    7.7930         0         0    7.0280];

qdot = zeros(9,1);
qdot = A*q_est+B*u;

== matlab function Time_Shift_1/Subsystem/state_NED_Obs ==
  data: state_NED input; state_NED_Obs output; P_NED_Obs input
function state_NED_Obs = fcn(state_NED,P_NED_Obs)
%#eml

state_NED_Obs = [P_NED_Obs(1);P_NED_Obs(2);P_NED_Obs(3);state_NED(4);state_NED(5);state_NED(6);state_NED(7);state_NED(8);...
    state_NED(9);state_NED(10);state_NED(11);state_NED(12);state_NED(13);state_NED(14);state_NED(15)];

== matlab function Time_Shift_1/Subsystem/Kalman_IC ==
  data: q_IC output
function q_IC = Kalman_IC()
%#eml
% 5000 Technology Dr., Huntsville AL 35899: 
% lon,lat,alt
%-86.647163*pi/180;34.718727*pi/180;195

% p_IC = -86.647163*pi/180;
% T_IC = 34.718727*pi/180;
% r_IC = 195;
% 
% P_ECNED_IC = ECFE2ECNED(p_IC,T_IC,r_IC);

% q_IC = [P_ECNED_IC(1);P_ECNED_IC(2);P_ECNED_IC(3);0;0;0;0;0;0];
q_IC = [0;0;0;0;0;0;0;0;0];

% end
% 
% function P_NED = ECFE2ECNED(p,T,r)
% % now apply projection matrix
% % p=state(1); % longitude
% % T=state(2); % lattitude
% % r=state(3); % Altitude
% 
% % ydot=state(7);
% % xdot=state(8);
% 
% % theta=pi/2-state(6);
% % thetap=-state(12);
% 
% R   = 6378.137e3;
% e_2 = 6.6943799014e-3;
% 
% NofT = R/sqrt(1-e_2*sin(T)^2);
% 
% X_ECFE=(r+NofT)*cos(T)*cos(p);
% Y_ECFE=(r+NofT)*cos(T)*sin(p);
% Z_ECFE=(r+NofT*(1-e_2))*sin(T);
% 
% R_ECFE_to_NED=[-sin(T)*cos(p) -sin(T)*sin(p) cos(T); -sin(p) cos(p) 0; -cos(T)*cos(p) -cos(T)*sin(p) -sin(T)];
% 
% P_ECFE =[X_ECFE;Y_ECFE;Z_ECFE];
% 
% P_NED=R_ECFE_to_NED*P_ECFE;
% end

== matlab function Time_Shift_1/Open-loop control/Camera Servos Function ==
  data: t input; PAN output; TILT output
function [PAN,TILT] = fcn(t)
%Insert Function for camera servo manipulation here
%By default, this function holds camera servos at their center position (1500 ms)
PAN = 1500;
TILT = 1500;

== matlab function Time_Shift_1/Open-loop control/plant/pulse transformer camera ==
  data: PAN input; TILT input; PAN_O output; TILT_O output
function [PAN_O, TILT_O]  = fcn(PAN,TILT)

PAN_O  = uint16(PAN);
TILT_O = uint16(TILT);

== matlab function Time_Shift_1/Sort for plotting ==
  data: longitude output; latitude output; altitude output; X output; Y output; Xe output; Ye output; dummy output; State_NED_Obs input; state_NED input; Qf input
function [longitude,latitude,altitude,X,Y,Xe,Ye,dummy]  = fcn(State_NED_Obs,state_NED,Qf)

%#codegen

% 
% %Note: NED = North direction(X), East direction(Y), Downward direction(Z)
%
% header = typecast(3908012345,'uint8');
% terminate = typecast(60532112345,'uint8');
longitude = typecast(Qf(1),'uint8');
latitude = typecast(Qf(2),'uint8');%latitude
altitude = typecast(Qf(3),'uint8'); %altitude
X = typecast(state_NED(1),'uint8'); %GPS provided X
Y = typecast(state_NED(2),'uint8');%GPS provided Y
%Z = typecast(state_NED(3),'uint8');%GPS provided Z

Xe = typecast(State_NED_Obs(1),'uint8');%Estimated X based on acceleration
Ye = typecast(State_NED_Obs(2),'uint8');%Estimated Y based on acceleration
%Ze = typecast(State_NED_Obs(3),'uint8');%Estimated Z based on acceleration
dummy = typecast(0,'uint8');

== matlab function Time_Shift_1/Open-loop control/plant/pulse transformer1 ==
  data: Left_PWM_I input; Right_PWM_I input; Left_PWM output; Right_PWM output
function [Left_PWM, Right_PWM]  = fcn(Left_PWM_I,Right_PWM_I)
% This block supports an embeddable subset of the MATLAB language.
% Converts output angle and speed value into a pulse width
% The input angle is between +pi/4 and -pi/4  (from limits)
% The speed is between 140 and 0 rps(Hz)

% angle=uint16(angI*16.25*180/pi + 1505.5);
% pw=-0.0002*speedI^3 +0.03*speedI^2 -2.66*speedI +1528;
% throtle = uint16(pw);
% 
Left_PWM  = uint16(Left_PWM_I);
Right_PWM = uint16(Right_PWM_I);

== matlab function Time_Shift_1/Status Extraction/Command State ==
  data: ID input; CCS output; byte input
function CCS = fcn(ID, byte)
% This block supports an embeddable subset of the MATLAB language.
% See the help menu for details. 
% outputs the command channel state (CCS) given status output

% first check that have proper status message
% ID = 10 for SSC status info
if ID==10
    if byte==2
        out=1;
    elseif byte==4;
        out=2;
    elseif byte==6
        out=3;
    else
        out=0;
    end
else
    out=4;
end
CCS = out;

== matlab function Time_Shift_1/status checker ==
  data: status input; enable output
function enable = fcn(status)
% This block supports an embeddable subset of the MATLAB language.
% See the help menu for details. 
if status==1  
    en = 1;
else
    en = -1;
end
enable=en;

== matlab function Time_Shift_1/Open-loop control/plant/Send Serial Packet to Servo Controller And recieve status message from SSC/Embedded MATLAB Function ==
  data: Packed input; CharArray output
function CharArray = fcn(Packed)
%
CharArray = zeros(22,1,'uint8');
CharArray = Packed;
